simulink model "planPublisher_test_RRT"  (R2020b)
settings: Solver=FixedStepAuto  StartTime=0.0  StopTime=inf  RelTol=1e-3
PreLoadFcn:
  | addpath('../ros_fun')
model workspace (MAT data in the model file):
  SL_ROS_VariableLengthArrays_MaxSizes.CommonInfo.ArrayTruncateAction = 'EmitWarning'
  SL_ROS_VariableLengthArrays_MaxSizes.MsgTypeMap = containers.Map
  SL_ROS_VariableLengthArrays_MaxSizes.MsgTypeMap.serialization.keys = {'nav_msgs/Path'}
  SL_ROS_VariableLengthArrays_MaxSizes.MsgTypeMap.serialization.values{1}.PropertyName = 'Poses'
  SL_ROS_VariableLengthArrays_MaxSizes.MsgTypeMap.serialization.values{1}.DataType = 'geometry_msgs/PoseStamped'
  SL_ROS_VariableLengthArrays_MaxSizes.MsgTypeMap.serialization.values{1}.MaxLength = 25
  SL_ROS_VariableLengthArrays_MaxSizes.MsgTypeMap.serialization.uniformity = 0
  SL_ROS_VariableLengthArrays_MaxSizes.MsgTypeMap.serialization.keyType = 'char'
  SL_ROS_VariableLengthArrays_MaxSizes.MsgTypeMap.serialization.valueType = 'any'
values from neighbouring files (symbols this model uses):
  desired_traj_RRT = zeros(size(pthObj.States,1),4)    [RRT.m]
libraries: robotlib x3
settings Model: Creator=bascetta  LastModifiedBy=root
settings OptimizationCC: EnhancedBackFolding=on  PassReuseOutputArgsAs=Individual arguments  ZeroExternalMemoryAtStartup=off  ZeroInternalMemoryAtStartup=off  MaxStackSize=64  OptimizeBlockOrder=speed  DifferentSizesBufferReuse=on  OptimizationCustomize=off  EfficientTunableParamExpr=on
settings DebuggingCC: ParameterTunabilityLossMsg=error
settings HardwareCC: ProdBitPerPointer=32  ProdBitPerSizeT=32  ProdBitPerPtrDiffT=32  ProdLargestAtomicFloat=None  ProdIntDivRoundTo=Undefined  ProdEndianess=Unspecified  ProdWordSize=32  ProdHWDeviceType=Generic->Unspecified (assume 32-bit Generic)
settings SFSimCC: MATLABDynamicMemAlloc=off  SimTargetLang=C++
settings RTWCC: Description=Embedded Coder  SystemTargetFile=ert.tlc  HardwareBoard=Robot Operating System (ROS)  TLCOptions="-aInlineSetEventsForThisBaseRateFcn=TLC_FALSE -aSuppressMultiTaskScheduler=TLC_FALSE  -aRateBasedStepFcn=0"  GenCodeOnly=on  TemplateMakefile=ert_default_tmf  Toolchain=Catkin  TargetLang=C++
settings CodeAppCC: ForceParamTrailComments=on  IgnoreCustomStorageClasses=off  OperatorAnnotations=on  SimulinkDataObjDesc=on  SFDataObjDesc=on  InsertBlockDesc=on
settings ERTTargetCC: SupportVariableSizeSignals=on  ERTCustomFileTemplate=rostime_codertarget_file_process.tlc

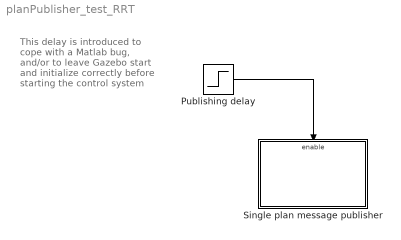
== system planPublisher_test_RRT ==
  note: This delay is introduced to cope with a Matlab bug,
      |  and/or to leave Gazebo start and initialize correctly before starting the control system
  Publishing delay : Step  Time=5
  Single plan message publisher : Subsystem
  wires:
  Publishing delay/1 -> Single plan message publisher/Enable

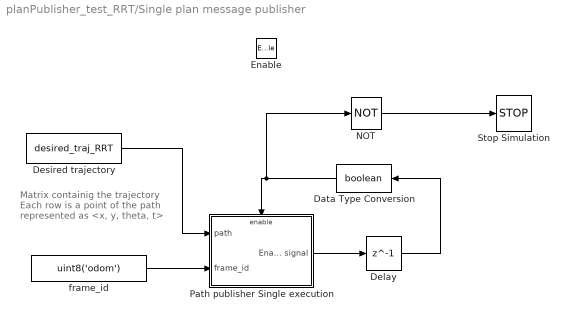
== system planPublisher_test_RRT/Single plan message publisher ==
  note: Matrix containig the trajectory
      | Each row is a point of the path
      | represented as <x, y, theta, t>
  Enable : EnablePort
  Data Type Conversion : DataTypeConversion  OutDataTypeStr=boolean  SaturateOnIntegerOverflow=on  RndMeth=Zero
  Delay : Delay  DelayLength=1  InitialCondition=1.0
  Desired trajectory : Constant  Value=desired_traj_RRT  VectorParams1D=off
  NOT : Logic  Operator=NOT  IconShape=distinctive  AllPortsSameDT=off  OutDataTypeStr=boolean
  Path publisher Single execution : Subsystem  TreatAsAtomicUnit=on
  Stop Simulation : Stop
  frame_id : Constant  Value=uint8('odom')
  wires:
  NOT/1 -> Stop Simulation/1
  Delay/1 -> Data Type Conversion/1
  frame_id/1 -> Path publisher Single execution/2(frame_id)
  Desired trajectory/1 -> Path publisher Single execution/1(path)
  Path publisher Single execution/1(Enable signal) -> Delay/1
  Data Type Conversion/1 -> NOT/1, Path publisher Single execution/Enable

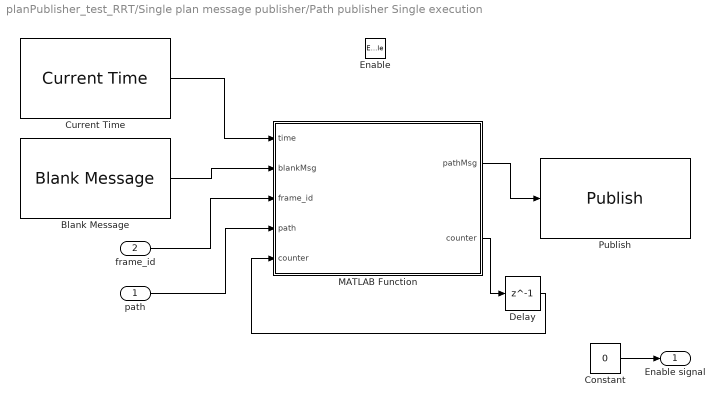
== system planPublisher_test_RRT/Single plan message publisher/Path publisher Single execution ==
  path : Inport
  frame_id : Inport  Port=2
  Enable : EnablePort
  Blank Message : robotlib/Blank Message  messageClass=Message  entityType=nav_msgs/Path  messageType=nav_msgs/Path  SampleTime=inf  legacyBusStruct=off
  Constant : Constant  Value=0
  Current Time : robotlib/Current Time  OutputFormat=double  SampleTime=-1  ModelName=planPublisher_test_RRT
      settings: SourceProductBaseCode=RR
  Delay : Delay  DelayLength=1  InitialCondition=0
  MATLAB Function : MATLAB Function  TreatAsAtomicUnit=on
  Publish : robotlib/Publish  topicSource=Specify your own  topic=/plan  messageType=nav_msgs/Path  legacyBusStruct=off  messageQueueLength=1
  Enable signal : Outport
  wires:
  Current Time/1 -> MATLAB Function/1(time)
  MATLAB Function/1(pathMsg) -> Publish/1
  path/1 -> MATLAB Function/4(path)
  frame_id/1 -> MATLAB Function/3(frame_id)
  Blank Message/1 -> MATLAB Function/2(blankMsg)
  Constant/1 -> Enable signal/1
  MATLAB Function/2(counter) -> Delay/1
  Delay/1 -> MATLAB Function/5("counter ")

== matlab function planPublisher_test_RRT/Single plan message publisher/Path publisher Single execution/MATLAB Function ==
  data: time input; blankMsg input; frame_id input; path input; pathMsg output Bus: SL_Bus_planPublisher_test_RRT_nav_msgs_Path; counter input; counter output
function [pathMsg,counter] = generate_path_msg(time,blankMsg,frame_id,path,counter)

len=min(25,size(path,1)-counter*25);

% Writing the message header
blankMsg.Header.Stamp.Sec = fix(time);
blankMsg.Header.Stamp.Nsec = fix((time-fix(time))*1e9);
blankMsg.Header.FrameId(1:length(frame_id)) = frame_id;
blankMsg.Header.FrameId_SL_Info.CurrentLength = uint32(length(frame_id));

% Set the number of poses
blankMsg.Poses_SL_Info.CurrentLength = uint32(len);
for seq=1:len
    pathPos=seq+25*counter;
    % Writing the header of each pose
    blankMsg.Poses(seq).Header.Stamp.Sec = fix(path(pathPos,4));
    blankMsg.Poses(seq).Header.Stamp.Nsec = fix((path(pathPos,4)-fix(path(pathPos,4)))*1e9);
    blankMsg.Poses(seq).Header.FrameId(1:length(frame_id)) = frame_id;
    blankMsg.Poses(seq).Header.FrameId_SL_Info.CurrentLength = uint32(length(frame_id));

    % Write pose data
    blankMsg.Poses(seq).Pose.Position.X = path(pathPos,1);
    blankMsg.Poses(seq).Pose.Position.Y = path(pathPos,2);
    blankMsg.Poses(seq).Pose.Position.Z = 0;
    
    orientation = eul2quat([0, 0, path(pathPos,3)], 'ZYX');
    blankMsg.Poses(seq).Pose.Orientation.X = orientation(1);
    blankMsg.Poses(seq).Pose.Orientation.Y = orientation(2);
    blankMsg.Poses(seq).Pose.Orientation.Z = orientation(3);
    blankMsg.Poses(seq).Pose.Orientation.W = orientation(4);
end
pathMsg = blankMsg;
counter=counter+1;
